simulink library "StateEstimation_lib"  (R2016b)
settings: Solver=VariableStepAuto  StartTime=0.0  StopTime=10.0  RelTol=1e-3
values from neighbouring files (symbols this model uses):
  accel_bias_init = zeros(3,1)    [Copy_of_StateEstimator_RIEKF.m]    (also in Quaternion_EKF.m; RightInvariant_EKF.m; StateEstimator_EKF.m; StateEstimator_RIEKF.m)
  accel_bias_noise_std = 0.1*ones(3,1)    [Copy_of_StateEstimator_RIEKF.m]    (also in Quaternion_EKF.m; RightInvariant_EKF.m; StateEstimator_EKF.m; StateEstimator_RIEKF.m)
  accel_noise_std = 0.1*ones(3,1)    [Copy_of_StateEstimator_RIEKF.m]    (also in Quaternion_EKF.m; RightInvariant_EKF.m; StateEstimator_EKF.m; StateEstimator_RIEKF.m)
  gyro_bias_init = zeros(3,1)    [Copy_of_StateEstimator_RIEKF.m]    (also in Quaternion_EKF.m; RightInvariant_EKF.m; StateEstimator_EKF.m; StateEstimator_RIEKF.m)
  gyro_bias_noise_std = 0.1*ones(3,1)    [Copy_of_StateEstimator_RIEKF.m]    (also in Quaternion_EKF.m; RightInvariant_EKF.m; StateEstimator_EKF.m; StateEstimator_RIEKF.m)
  gyro_noise_std = 0.1*ones(3,1)    [Copy_of_StateEstimator_RIEKF.m]    (also in Quaternion_EKF.m; RightInvariant_EKF.m; StateEstimator_EKF.m; StateEstimator_RIEKF.m)
undefined symbols (not defined in the file or in its folder): cassieParameters, CassieParameters, EKF_SampleTime, q_init, v_init
libraries: xpcutilitieslib x41, xpcrtudplib x41, dspfdesign x10, simulink x6, slrtlib x5
(part 2 of 4)

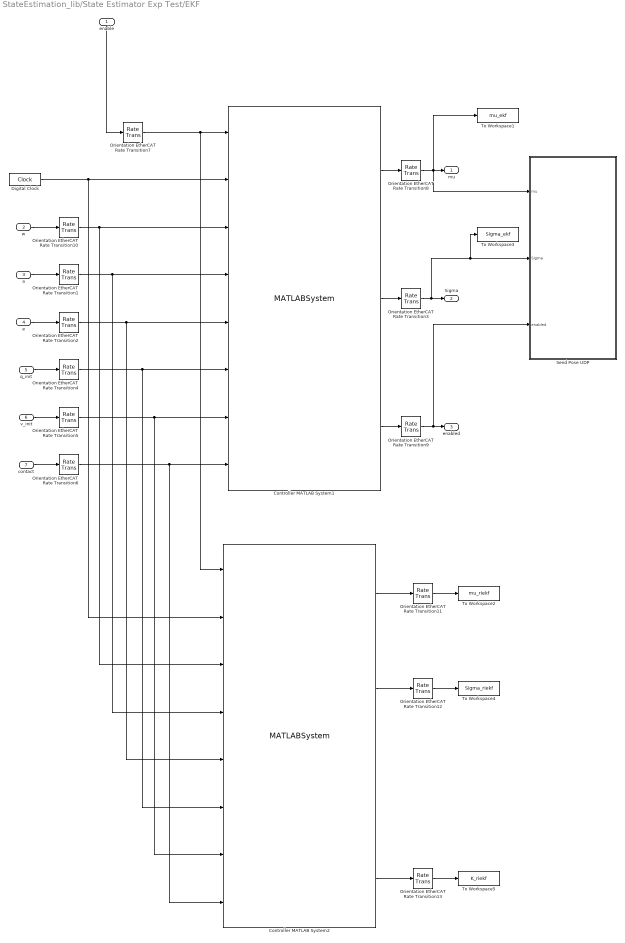
== system StateEstimation_lib/State Estimator Exp Test/EKF ==
  enable : Inport
  w : Inport  Port=2
  a : Inport  Port=3
  e : Inport  Port=4
  q_init : Inport  Port=5
  v_init : Inport  Port=6
  contact : Inport  Port=7
  Controller MATLAB System1 : MATLABSystem  System=StateEstimator_EKF  static_bias_initialization=static_bias_initialization  ekf_update_enabled=true  dt=EKF_SampleTime  enable_bias_estimation=enable_bias_estimation  gyro_noise_std=gyro_noise_std  gyro_bias_noise_std=gyro_bias_noise_std  accel_noise_std=accel_noise_std  accel_bias_noise_std=accel_bias_noise_std  contact_noise_std=contact_noise_std  encoder_noise_std=encoder_noise_std  gyro_bias_init=gyro_bias_init  accel_bias_init=accel_bias_init  SimulateUsing=Code generation
      mask Type: StateEstimator_EKF
      mask Display:
      | disp('StateEstimator_EKF');
      | port_label('input',1,'EnableFilter');
      | port_label('input',2,'t');
      | port_label('input',3,'w');
      | port_label('input',4,'a');
      | port_label('input',5,'e');
      | port_label('input',6,'q_init');
      | port_label('input',7,'v_init');
      | port_label('input',8,'contact');
      | port_label('output',1,'mu');
      | port_label('output',2,'Sigma');
      | port_label('output',3,'enabled');
  Controller MATLAB System2 : MATLABSystem  System=StateEstimator_RIEKF  static_bias_initialization=static_bias_initialization  ekf_update_enabled=true  dt=EKF_SampleTime  enable_bias_estimation=enable_bias_estimation  gyro_noise_std=gyro_noise_std  gyro_bias_noise_std=gyro_bias_noise_std  accel_noise_std=accel_noise_std  accel_bias_noise_std=accel_bias_noise_std  contact_noise_std=contact_noise_std  encoder_noise_std=encoder_noise_std  gyro_bias_init=gyro_bias_init  accel_bias_init=accel_bias_init  SimulateUsing=Code generation
      mask Type: StateEstimator_RIEKF
      mask Display:
      | disp('StateEstimator_RIEKF');
      | port_label('input',1,'EnableFilter');
      | port_label('input',2,'t');
      | port_label('input',3,'w');
      | port_label('input',4,'a');
      | port_label('input',5,'e');
      | port_label('input',6,'q_init');
      | port_label('input',7,'v_init');
      | port_label('input',8,'contact');
      | port_label('output',1,'mu');
      | port_label('output',2,'Sigma');
      | port_label('output',3,'enabled');
      | port_label('output',4,'K');
  Digital Clock : DigitalClock  SampleTime=EKF_SampleTime
  Orientation EtherCAT Rate Transition{1..2,4..7,10} (7 alike) : RateTransition  Deterministic=off  OutPortSampleTime=EKF_SampleTime
  Orientation EtherCAT Rate Transition{3,8..9,11..13} (6 alike) : RateTransition  Deterministic=off  OutPortSampleTime=CassieParameters.etherCatSampleTime
  Send Pose UDP : Subsystem
  To Workspace1 : ToWorkspace  VariableName=mu_ekf  SaveFormat=Timeseries  SampleTime=-1
  To Workspace2 : ToWorkspace  VariableName=mu_riekf  SaveFormat=Timeseries  SampleTime=-1
  To Workspace3 : ToWorkspace  VariableName=Sigma_ekf  SaveFormat=Timeseries  SampleTime=-1
  To Workspace4 : ToWorkspace  VariableName=Sigma_riekf  SaveFormat=Timeseries  SampleTime=-1
  To Workspace5 : ToWorkspace  VariableName=K_riekf  SaveFormat=Timeseries  SampleTime=-1
  mu : Outport
  Sigma : Outport  Port=2
  enabled : Outport  Port=3
  wires:
  enable/1 -> Orientation EtherCAT Rate Transition7/1
  Orientation EtherCAT Rate Transition7/1 -> Controller MATLAB System2/1, Controller MATLAB System1/1
  Orientation EtherCAT Rate Transition8/1 -> To Workspace1/1, Send Pose UDP/1(mu), mu/1
  Digital Clock/1 -> Controller MATLAB System2/2, Controller MATLAB System1/2
  Orientation EtherCAT Rate Transition9/1 -> Send Pose UDP/3(enabled), enabled/1
  Controller MATLAB System1/1 -> Orientation EtherCAT Rate Transition8/1
  Controller MATLAB System1/3 -> Orientation EtherCAT Rate Transition9/1
  Orientation EtherCAT Rate Transition6/1 -> Controller MATLAB System2/8, Controller MATLAB System1/8
  Orientation EtherCAT Rate Transition5/1 -> Controller MATLAB System2/7, Controller MATLAB System1/7
  q_init/1 -> Orientation EtherCAT Rate Transition4/1
  v_init/1 -> Orientation EtherCAT Rate Transition5/1
  contact/1 -> Orientation EtherCAT Rate Transition6/1
  w/1 -> Orientation EtherCAT Rate Transition10/1
  Orientation EtherCAT Rate Transition10/1 -> Controller MATLAB System2/3, Controller MATLAB System1/3
  a/1 -> Orientation EtherCAT Rate Transition1/1
  e/1 -> Orientation EtherCAT Rate Transition2/1
  Controller MATLAB System1/2 -> Orientation EtherCAT Rate Transition3/1
  Orientation EtherCAT Rate Transition3/1 -> To Workspace3/1, Send Pose UDP/2(Sigma), Sigma/1
  Orientation EtherCAT Rate Transition1/1 -> Controller MATLAB System2/4, Controller MATLAB System1/4
  Orientation EtherCAT Rate Transition2/1 -> Controller MATLAB System2/5, Controller MATLAB System1/5
  Orientation EtherCAT Rate Transition4/1 -> Controller MATLAB System2/6, Controller MATLAB System1/6
  Controller MATLAB System2/1 -> Orientation EtherCAT Rate Transition11/1
  Orientation EtherCAT Rate Transition11/1 -> To Workspace2/1
  Controller MATLAB System2/2 -> Orientation EtherCAT Rate Transition12/1
  Orientation EtherCAT Rate Transition12/1 -> To Workspace4/1
  Controller MATLAB System2/4 -> Orientation EtherCAT Rate Transition13/1
  Orientation EtherCAT Rate Transition13/1 -> To Workspace5/1

== system StateEstimation_lib/State Estimator Exp Test/Kinematic Velocity Estimator ==
  w : Inport
  q : Inport  Port=2
  dq : Inport  Port=3
  contact : Inport  Port=4
  Kinematic_Velocity : MATLAB Function  TreatAsAtomicUnit=on
  Selector2 : Selector  InputPortWidth=20  IndexOptions=Index vector (dialog)  Indices=[7:20]  OutputSizes=1
  Selector3 : Selector  InputPortWidth=20  IndexOptions=Index vector (dialog)  Indices=[7:20]  OutputSizes=1
  velocity_kinematic : Outport
  wires:
  w/1 -> Kinematic_Velocity/1(w)
  contact/1 -> Kinematic_Velocity/4(contact)
  dq/1 -> Selector3/1
  Kinematic_Velocity/1(velocity) -> velocity_kinematic/1
  q/1 -> Selector2/1
  Selector3/1 -> Kinematic_Velocity/3(e_dot)
  Selector2/1 -> Kinematic_Velocity/2(e)

== system StateEstimation_lib/State Estimator Exp Test/Local Map UDP ==
  note: Local Map UDP Data Structure
      |
      | Map Information
      | double time
      | double resolution
      | double length_x
      | double length_y
      |
      | Map Center Pose
      | double position_x
      | double position_y
      | double position_z
      | double orientation_x
      | double orientation_y
      | double orientation_z
      | double orientation_w
      |
      | Update Block Data
      | double row_start_index
      | double column_start_index
      | double[100] elevation_data
  "Byte Unpacking " : xpcutilitieslib/Byte Unpacking   MaskUnpackedDataTypes={'double'}  MaskUnpackedDataSizes={[45]}  MaskAlignment=1
  Data Store Memory : DataStoreMemory  DataStoreName=local_map  ReadBeforeWriteMsg=warning  WriteAfterWriteMsg=warning  WriteAfterReadMsg=warning  ShowAdditionalParam=off
  Data Store Write : DataStoreWrite  DataStoreName=local_map
  Receive : xpcrtudplib/UDP Receive  ipAddressVal=Use host-target connection  localPort=25000  rcvWidth=45*8  rcvFmAny=off  fmAddress=10.10.10.5  sampleTime=-1
  Terminator : Terminator
  wires:
  Receive/2 -> Terminator/1
  Receive/1 -> "Byte Unpacking "/1
  "Byte Unpacking "/1 -> Data Store Write/1

== system StateEstimation_lib/State Estimator Exp Test/Parse Outputs ==
  outputs : Inport
  Bus Selector : BusSelector  OutputSignals=radio
  Parse_Outputs : MATLAB Function  TreatAsAtomicUnit=on
  Send IMU UDP : Subsystem
  Send JointState UDP : Subsystem
  Send Radio : Subsystem
  Send Time : Subsystem
  qwi : Outport
  wi : Outport  Port=2
  ai : Outport  Port=3
  q : Outport  Port=4
  dq : Outport  Port=5
  wires:
  Bus Selector/1 -> Send Radio/1(radio)  "<radio>"
  Parse_Outputs/5(dq) -> dq/1, Send JointState UDP/2(dq)
  outputs/1 -> Bus Selector/1, Parse_Outputs/1(outputs)
  Parse_Outputs/2(wi) -> Send IMU UDP/2(w), wi/1
  Parse_Outputs/4(q) -> q/1, Send JointState UDP/1(q)
  Parse_Outputs/1(qwi) -> qwi/1, Send IMU UDP/1(q)
  Parse_Outputs/3(ai) -> Send IMU UDP/3(a), ai/1

== system StateEstimation_lib/State Estimator Exp Test/Reconstruct State ==
  q_in : Inport
  dq_in : Inport  Port=2
  w : Inport  Port=3
  contact : Inport  Port=4
  mu_in : Inport  Port=5
  ekf_enabled : Inport  Port=6
  Construct_State : MATLAB Function  TreatAsAtomicUnit=on
  Low Pass Filter : Subsystem  TreatAsAtomicUnit=on
  Mux : Mux
  Scope 6 : slrtlib/Displays and Logging/Scope   scopeno=2  scopetype=File  autostart=on  viewmode=Numerical  formatstr='%15.6f'  grid=on  ylimits=[0,0]  nosamples=250  noprepostsamples=0  interleave=1  triggermode=FreeRun  triggersignal=1  trigsignalfromport=on  triggerlevel=0.5  triggerslope=Rising  triggerscope=1  triggersample=0  filename=ekf1.dat  mode=Commit  writesize=512  autorestart=on  dynamicfilemode=off  maxwritefilesize=4000*1024^2
  q : Outport
  dq : Outport  Port=2
  velocity : Outport  Port=3
  wires:
  Low Pass Filter/1(filtered_signal) -> velocity/1
  mu_in/1 -> Construct_State/5(mu), Mux/3
  dq_in/1 -> Construct_State/2("dq ")
  Construct_State/1(q) -> q/1
  Construct_State/3(velocity) -> Mux/1, Low Pass Filter/1(signal)
  Construct_State/5(filter_selector) -> Low Pass Filter/2(selector)
  Mux/1 -> Scope 6/1
  q_in/1 -> Construct_State/1("q ")
  ekf_enabled/1 -> Construct_State/6(ekf_enabled), Mux/4
  Construct_State/2(dq) -> dq/1
  w/1 -> Construct_State/3(w)
  contact/1 -> Construct_State/4(contact)
  Construct_State/4(velocity_kinematic) -> Mux/2

== system StateEstimation_lib/State Estimator Sim Test/Contact Estimator ==
  q : Inport
  GRF_Estimator : MATLAB Function  TreatAsAtomicUnit=on
  Selector : Selector  InputPortWidth=4  IndexOptions=Index vector (dialog)  Indices=[2, 4]  OutputSizes=1
  Send Contact : Subsystem
  GRF : Outport
  contact : Outport  Port=2
  wires:
  GRF_Estimator/1(GRF) -> Selector/1, GRF/1
  GRF_Estimator/2(contact) -> contact/1
  q/1 -> GRF_Estimator/1(q)
  Selector/1 -> Send Contact/1(contact)

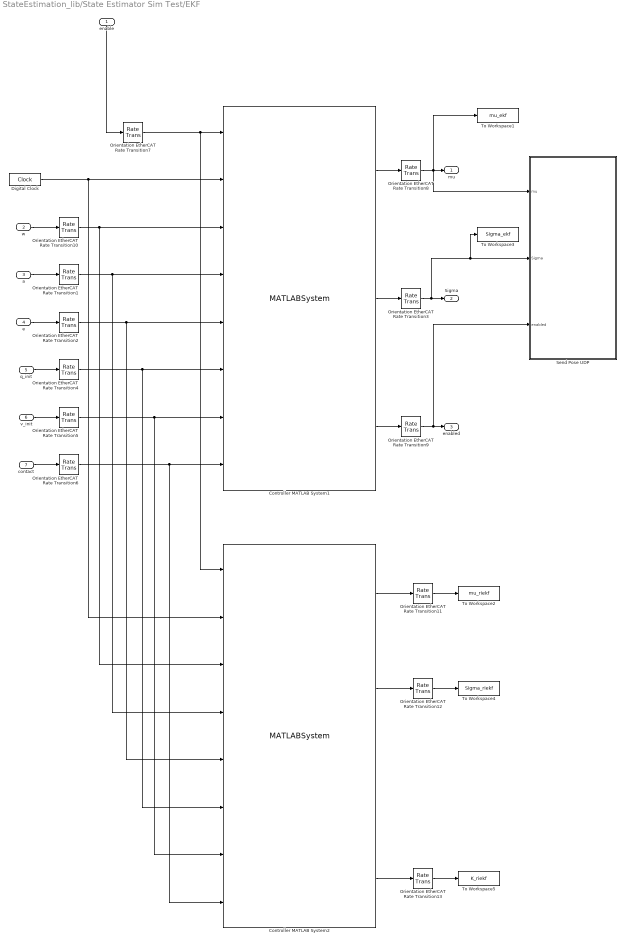
== system StateEstimation_lib/State Estimator Sim Test/EKF ==
  enable : Inport
  w : Inport  Port=2
  a : Inport  Port=3
  e : Inport  Port=4
  q_init : Inport  Port=5
  v_init : Inport  Port=6
  contact : Inport  Port=7
  Controller MATLAB System1 : MATLABSystem  System=StateEstimator_EKF  static_bias_initialization=true  ekf_update_enabled=true  dt=EKF_SampleTime  enable_bias_estimation=enable_bias_estimation  gyro_noise_std=gyro_noise_std  gyro_bias_noise_std=gyro_bias_noise_std  accel_noise_std=accel_noise_std  accel_bias_noise_std=accel_bias_noise_std  contact_noise_std=contact_noise_std  encoder_noise_std=encoder_noise_std  gyro_bias_init=[0;0;0]  accel_bias_init=[0;0;0]  SimulateUsing=Interpreted execution
      mask Type: StateEstimator_EKF
      mask Display:
      | disp('StateEstimator_EKF');
      | port_label('input',1,'EnableFilter');
      | port_label('input',2,'t');
      | port_label('input',3,'w');
      | port_label('input',4,'a');
      | port_label('input',5,'e');
      | port_label('input',6,'q_init');
      | port_label('input',7,'v_init');
      | port_label('input',8,'contact');
      | port_label('output',1,'mu');
      | port_label('output',2,'Sigma');
      | port_label('output',3,'enabled');
  Controller MATLAB System2 : MATLABSystem  System=StateEstimator_RIEKF  static_bias_initialization=true  ekf_update_enabled=true  dt=EKF_SampleTime  enable_bias_estimation=enable_bias_estimation  gyro_noise_std=gyro_noise_std  gyro_bias_noise_std=gyro_bias_noise_std  accel_noise_std=accel_noise_std  accel_bias_noise_std=accel_bias_noise_std  contact_noise_std=contact_noise_std  encoder_noise_std=encoder_noise_std  gyro_bias_init=[0;0;0]  accel_bias_init=[0;0;0]  SimulateUsing=Code generation
      mask Type: StateEstimator_RIEKF
      mask Display:
      | disp('StateEstimator_RIEKF');
      | port_label('input',1,'EnableFilter');
      | port_label('input',2,'t');
      | port_label('input',3,'w');
      | port_label('input',4,'a');
      | port_label('input',5,'e');
      | port_label('input',6,'q_init');
      | port_label('input',7,'v_init');
      | port_label('input',8,'contact');
      | port_label('output',1,'mu');
      | port_label('output',2,'Sigma');
      | port_label('output',3,'enabled');
      | port_label('output',4,'K');
  Digital Clock : DigitalClock  SampleTime=EKF_SampleTime
  Orientation EtherCAT Rate Transition{1..2,4..7,10} (7 alike) : RateTransition  Deterministic=off  OutPortSampleTime=EKF_SampleTime
  Orientation EtherCAT Rate Transition{3,8..9,11..13} (6 alike) : RateTransition  Deterministic=off  OutPortSampleTime=CassieParameters.etherCatSampleTime
  Send Pose UDP : Subsystem
  To Workspace1 : ToWorkspace  VariableName=mu_ekf  SaveFormat=Timeseries  SampleTime=-1
  To Workspace2 : ToWorkspace  VariableName=mu_riekf  SaveFormat=Timeseries  SampleTime=-1
  To Workspace3 : ToWorkspace  VariableName=Sigma_ekf  SaveFormat=Timeseries  SampleTime=-1
  To Workspace4 : ToWorkspace  VariableName=Sigma_riekf  SaveFormat=Timeseries  SampleTime=-1
  To Workspace5 : ToWorkspace  VariableName=K_riekf  SaveFormat=Timeseries  SampleTime=-1
  mu : Outport
  Sigma : Outport  Port=2
  enabled : Outport  Port=3
  wires:
  enable/1 -> Orientation EtherCAT Rate Transition7/1
  Orientation EtherCAT Rate Transition7/1 -> Controller MATLAB System2/1, Controller MATLAB System1/1
  Orientation EtherCAT Rate Transition8/1 -> To Workspace1/1, Send Pose UDP/1(mu), mu/1
  Digital Clock/1 -> Controller MATLAB System2/2, Controller MATLAB System1/2
  Orientation EtherCAT Rate Transition9/1 -> Send Pose UDP/3(enabled), enabled/1
  Controller MATLAB System1/1 -> Orientation EtherCAT Rate Transition8/1
  Controller MATLAB System1/3 -> Orientation EtherCAT Rate Transition9/1
  Orientation EtherCAT Rate Transition6/1 -> Controller MATLAB System2/8, Controller MATLAB System1/8
  Orientation EtherCAT Rate Transition5/1 -> Controller MATLAB System2/7, Controller MATLAB System1/7
  q_init/1 -> Orientation EtherCAT Rate Transition4/1
  v_init/1 -> Orientation EtherCAT Rate Transition5/1
  contact/1 -> Orientation EtherCAT Rate Transition6/1
  w/1 -> Orientation EtherCAT Rate Transition10/1
  Orientation EtherCAT Rate Transition10/1 -> Controller MATLAB System2/3, Controller MATLAB System1/3
  a/1 -> Orientation EtherCAT Rate Transition1/1
  e/1 -> Orientation EtherCAT Rate Transition2/1
  Controller MATLAB System1/2 -> Orientation EtherCAT Rate Transition3/1
  Orientation EtherCAT Rate Transition3/1 -> To Workspace3/1, Send Pose UDP/2(Sigma), Sigma/1
  Orientation EtherCAT Rate Transition1/1 -> Controller MATLAB System2/4, Controller MATLAB System1/4
  Orientation EtherCAT Rate Transition2/1 -> Controller MATLAB System2/5, Controller MATLAB System1/5
  Orientation EtherCAT Rate Transition4/1 -> Controller MATLAB System2/6, Controller MATLAB System1/6
  Controller MATLAB System2/1 -> Orientation EtherCAT Rate Transition11/1
  Orientation EtherCAT Rate Transition11/1 -> To Workspace2/1
  Controller MATLAB System2/2 -> Orientation EtherCAT Rate Transition12/1
  Orientation EtherCAT Rate Transition12/1 -> To Workspace4/1
  Controller MATLAB System2/4 -> Orientation EtherCAT Rate Transition13/1
  Orientation EtherCAT Rate Transition13/1 -> To Workspace5/1

== system StateEstimation_lib/State Estimator Sim Test/Kinematic Velocity Estimator ==
  w : Inport
  q : Inport  Port=2
  dq : Inport  Port=3
  contact : Inport  Port=4
  Kinematic_Velocity : MATLAB Function  TreatAsAtomicUnit=on
  Selector2 : Selector  InputPortWidth=20  IndexOptions=Index vector (dialog)  Indices=[7:20]  OutputSizes=1
  Selector3 : Selector  InputPortWidth=20  IndexOptions=Index vector (dialog)  Indices=[7:20]  OutputSizes=1
  velocity_kinematic : Outport
  wires:
  w/1 -> Kinematic_Velocity/1(w)
  contact/1 -> Kinematic_Velocity/4(contact)
  dq/1 -> Selector3/1
  Kinematic_Velocity/1(velocity) -> velocity_kinematic/1
  q/1 -> Selector2/1
  Selector3/1 -> Kinematic_Velocity/3(e_dot)
  Selector2/1 -> Kinematic_Velocity/2(e)

== system StateEstimation_lib/State Estimator Sim Test/Local Map UDP ==
  note: Local Map UDP Data Structure
      |
      | Map Information
      | double time
      | double resolution
      | double length_x
      | double length_y
      |
      | Map Center Pose
      | double position_x
      | double position_y
      | double position_z
      | double orientation_x
      | double orientation_y
      | double orientation_z
      | double orientation_w
      |
      | Update Block Data
      | double row_start_index
      | double column_start_index
      | double[100] elevation_data
  "Byte Unpacking " : xpcutilitieslib/Byte Unpacking   MaskUnpackedDataTypes={'double'}  MaskUnpackedDataSizes={[45]}  MaskAlignment=1
  Data Store Memory : DataStoreMemory  DataStoreName=local_map  ReadBeforeWriteMsg=warning  WriteAfterWriteMsg=warning  WriteAfterReadMsg=warning  ShowAdditionalParam=off
  Data Store Write : DataStoreWrite  DataStoreName=local_map
  Receive : xpcrtudplib/UDP Receive  ipAddressVal=Use host-target connection  localPort=25000  rcvWidth=45*8  rcvFmAny=off  fmAddress=10.10.10.5  sampleTime=-1
  Terminator : Terminator
  wires:
  Receive/2 -> Terminator/1
  Receive/1 -> "Byte Unpacking "/1
  "Byte Unpacking "/1 -> Data Store Write/1

== system StateEstimation_lib/State Estimator Sim Test/Parse Outputs ==
  outputs : Inport
  Bus Selector : BusSelector  OutputSignals=radio
  Parse_Outputs : MATLAB Function  TreatAsAtomicUnit=on
  Send IMU UDP : Subsystem
  Send JointState UDP : Subsystem
  Send Radio : Subsystem
  Send Time : Subsystem
  qwi : Outport
  wi : Outport  Port=2
  ai : Outport  Port=3
  q : Outport  Port=4
  dq : Outport  Port=5
  wires:
  Bus Selector/1 -> Send Radio/1(radio)  "<radio>"
  Parse_Outputs/5(dq) -> dq/1, Send JointState UDP/2(dq)
  outputs/1 -> Bus Selector/1, Parse_Outputs/1(outputs)
  Parse_Outputs/2(wi) -> Send IMU UDP/2(w), wi/1
  Parse_Outputs/4(q) -> q/1, Send JointState UDP/1(q)
  Parse_Outputs/1(qwi) -> qwi/1, Send IMU UDP/1(q)
  Parse_Outputs/3(ai) -> Send IMU UDP/3(a), ai/1

== system StateEstimation_lib/State Estimator Sim Test/Reconstruct State ==
  q_in : Inport
  dq_in : Inport  Port=2
  w : Inport  Port=3
  contact : Inport  Port=4
  mu_in : Inport  Port=5
  ekf_enabled : Inport  Port=6
  Construct_State : MATLAB Function  TreatAsAtomicUnit=on
  Low Pass Filter : Subsystem  TreatAsAtomicUnit=on
  Mux : Mux
  Scope 6 : slrtlib/Displays and Logging/Scope   scopeno=1  scopetype=File  autostart=on  viewmode=Numerical  formatstr='%15.6f'  grid=on  ylimits=[0,0]  nosamples=250  noprepostsamples=0  interleave=1  triggermode=FreeRun  triggersignal=1  trigsignalfromport=on  triggerlevel=0.5  triggerslope=Rising  triggerscope=1  triggersample=0  filename=ekf.dat  mode=Commit  writesize=512  autorestart=on  dynamicfilemode=off  maxwritefilesize=4000*1024^2
  q : Outport
  dq : Outport  Port=2
  velocity : Outport  Port=3
  wires:
  Low Pass Filter/1(filtered_signal) -> velocity/1
  mu_in/1 -> Construct_State/5(mu), Mux/3
  dq_in/1 -> Construct_State/2("dq ")
  Construct_State/1(q) -> q/1
  Construct_State/3(velocity) -> Mux/1, Low Pass Filter/1(signal)
  Construct_State/5(filter_selector) -> Low Pass Filter/2(selector)
  Mux/1 -> Scope 6/1
  q_in/1 -> Construct_State/1("q ")
  ekf_enabled/1 -> Construct_State/6(ekf_enabled), Mux/4
  Construct_State/2(dq) -> dq/1
  w/1 -> Construct_State/3(w)
  contact/1 -> Construct_State/4(contact)
  Construct_State/4(velocity_kinematic) -> Mux/2

== system StateEstimation_lib/Quaternion-based EKF/Contact Estimator/Send Contact ==
  contact : Inport
  "Byte Packing " : xpcutilitieslib/Byte Packing   MaskPackedDataType=uint8  MaskUnpackedDataTypes={'double'}  MaskAlignment=1
  Digital Clock : DigitalClock  SampleTime=CassieParameters.etherCatSampleTime
  Mux1 : Mux  Inputs=2
  Orientation EtherCAT Rate Transition10 : RateTransition  Deterministic=off  OutPortSampleTime=Contact_UDP_SampleTime
  Send : xpcrtudplib/UDP Send  ipAddressVal=Use host-target connection  localPort=-1  toAddress=10.10.10.5  toPort=25004  sampleTime=Contact_UDP_SampleTime
  Width : Width
  wires:
  Mux1/1 -> Orientation EtherCAT Rate Transition10/1
  "Byte Packing "/1 -> Width/1, Send/1
  Width/1 -> Send/2
  Orientation EtherCAT Rate Transition10/1 -> "Byte Packing "/1
  Digital Clock/1 -> Mux1/1
  contact/1 -> Mux1/2

== system StateEstimation_lib/Quaternion-based EKF/EKF/Send Pose UDP ==
  mu : Inport
  Sigma : Inport  Port=2
  enabled : Inport  Port=3
  "Byte Packing " : xpcutilitieslib/Byte Packing   MaskPackedDataType=uint8  MaskUnpackedDataTypes={'double'}  MaskAlignment=1
  ConstructPoseData : MATLAB Function  TreatAsAtomicUnit=on
  Digital Clock : DigitalClock  SampleTime=CassieParameters.etherCatSampleTime
  Mux1 : Mux
  Orientation EtherCAT Rate Transition10 : RateTransition  Deterministic=off  OutPortSampleTime=Pose_UDP_SampleTime
  Send : xpcrtudplib/UDP Send  ipAddressVal=Use host-target connection  localPort=-1  toAddress=10.10.10.5  toPort=25000  sampleTime=Pose_UDP_SampleTime
  Width : Width
  wires:
  Mux1/1 -> Orientation EtherCAT Rate Transition10/1
  "Byte Packing "/1 -> Width/1, Send/1
  Width/1 -> Send/2
  Orientation EtherCAT Rate Transition10/1 -> "Byte Packing "/1
  mu/1 -> Mux1/4, ConstructPoseData/1(mu)
  Sigma/1 -> ConstructPoseData/2(Sigma)
  enabled/1 -> Mux1/2
  Digital Clock/1 -> Mux1/1
  ConstructPoseData/1(pose_data) -> Mux1/3

== system StateEstimation_lib/Quaternion-based EKF/Parse Outputs/Send IMU UDP ==
  q : Inport
  w : Inport  Port=2
  a : Inport  Port=3
  "Byte Packing " : xpcutilitieslib/Byte Packing   MaskPackedDataType=uint8  MaskUnpackedDataTypes={'double'}  MaskAlignment=1
  Digital Clock : DigitalClock  SampleTime=CassieParameters.etherCatSampleTime
  Invert Quaterion for ROS : MATLAB Function  TreatAsAtomicUnit=on
  Mux1 : Mux
  Orientation EtherCAT Rate Transition10 : RateTransition  Deterministic=off  OutPortSampleTime=IMU_UDP_SampleTime
  Send : xpcrtudplib/UDP Send  ipAddressVal=Use host-target connection  localPort=-1  toAddress=10.10.10.5  toPort=25001  sampleTime=IMU_UDP_SampleTime
  Width : Width
  wires:
  Mux1/1 -> Orientation EtherCAT Rate Transition10/1
  "Byte Packing "/1 -> Width/1, Send/1
  Width/1 -> Send/2
  Orientation EtherCAT Rate Transition10/1 -> "Byte Packing "/1
  Digital Clock/1 -> Mux1/1
  a/1 -> Mux1/4
  q/1 -> Invert Quaterion for ROS/1(q)
  w/1 -> Mux1/3
  Invert Quaterion for ROS/1(q_inv) -> Mux1/2

== system StateEstimation_lib/Quaternion-based EKF/Parse Outputs/Send JointState UDP ==
  q : Inport
  dq : Inport  Port=2
  "Byte Packing " : xpcutilitieslib/Byte Packing   MaskPackedDataType=uint8  MaskUnpackedDataTypes={'double'}  MaskAlignment=1
  Digital Clock : DigitalClock  SampleTime=CassieParameters.etherCatSampleTime
  Mux1 : Mux  Inputs=3
  Orientation EtherCAT Rate Transition10 : RateTransition  Deterministic=off  OutPortSampleTime=JointState_UDP_SampleTime
  Parse_Outputs : MATLAB Function  TreatAsAtomicUnit=on
  Send : xpcrtudplib/UDP Send  ipAddressVal=Use host-target connection  localPort=-1  toAddress=10.10.10.5  toPort=25002  sampleTime=JointState_UDP_SampleTime
  Width : Width
  wires:
  Mux1/1 -> Orientation EtherCAT Rate Transition10/1
  "Byte Packing "/1 -> Width/1, Send/1
  Width/1 -> Send/2
  Orientation EtherCAT Rate Transition10/1 -> "Byte Packing "/1
  Digital Clock/1 -> Mux1/1
  Parse_Outputs/1(q_reduced) -> Mux1/2
  Parse_Outputs/2(dq_reduced) -> Mux1/3
  dq/1 -> Parse_Outputs/2(dq)
  q/1 -> Parse_Outputs/1(q)

== system StateEstimation_lib/Quaternion-based EKF/Parse Outputs/Send Radio ==
  radio : Inport
  "Byte Packing " : xpcutilitieslib/Byte Packing   MaskPackedDataType=uint8  MaskUnpackedDataTypes={'double'}  MaskAlignment=1
  Digital Clock : DigitalClock  SampleTime=CassieParameters.etherCatSampleTime
  Mux1 : Mux  Inputs=2
  Orientation EtherCAT Rate Transition10 : RateTransition  Deterministic=off  OutPortSampleTime=Radio_UDP_SampleTime
  Send : xpcrtudplib/UDP Send  ipAddressVal=Use host-target connection  localPort=-1  toAddress=10.10.10.5  toPort=25003  sampleTime=Radio_UDP_SampleTime
  Width : Width
  wires:
  Mux1/1 -> Orientation EtherCAT Rate Transition10/1
  "Byte Packing "/1 -> Width/1, Send/1
  Width/1 -> Send/2
  Orientation EtherCAT Rate Transition10/1 -> "Byte Packing "/1
  Digital Clock/1 -> Mux1/1
  radio/1 -> Mux1/2

== system StateEstimation_lib/Quaternion-based EKF/Parse Outputs/Send Time ==
  "Byte Packing " : xpcutilitieslib/Byte Packing   MaskPackedDataType=uint8  MaskUnpackedDataTypes={'double'}  MaskAlignment=1
  Digital Clock : DigitalClock  SampleTime=CassieParameters.etherCatSampleTime
  Orientation EtherCAT Rate Transition10 : RateTransition  Deterministic=off  OutPortSampleTime=Time_UDP_SampleTime
  Send : xpcrtudplib/UDP Send  ipAddressVal=Use host-target connection  localPort=-1  toAddress=10.10.10.105  toPort=25005  sampleTime=Time_UDP_SampleTime
  Width : Width
  wires:
  Digital Clock/1 -> Orientation EtherCAT Rate Transition10/1
  "Byte Packing "/1 -> Width/1, Send/1
  Width/1 -> Send/2
  Orientation EtherCAT Rate Transition10/1 -> "Byte Packing "/1

== system StateEstimation_lib/Quaternion-based EKF/Reconstruct State/Low Pass Filter ==
  signal : Inport  Partition=on  PartitionDimension=1  PartitionWidth=1
  selector : Inport  Port=2
  For Each : ForEach  DisableCoverage=on  IndexMode=One-based
  Lowpass Filter : dspfdesign/Lowpass Filter  FilterType=FIR  DesignForMinimumOrder=on  FilterOrder=50  PassbandFrequency=1  StopbandFrequency=10  PassbandRipple=1  StopbandAttenuation=20  InheritSampleRate=off  SampleRate=2000  SimulateUsing=Code generation  roundingMode=Floor  coeffsDataTypeStr=fixdt(1,16)
  Lowpass Filter1 : dspfdesign/Lowpass Filter  FilterType=FIR  DesignForMinimumOrder=on  FilterOrder=50  PassbandFrequency=1  StopbandFrequency=5  PassbandRipple=1  StopbandAttenuation=30  InheritSampleRate=off  SampleRate=2000  SimulateUsing=Code generation  roundingMode=Floor  coeffsDataTypeStr=fixdt(1,16)
  Switch : Switch  Criteria=u2 > Threshold
  filtered_signal : Outport  ConcatenationDimension=1
  wires:
  signal/1 -> Lowpass Filter1/1, Lowpass Filter/1
  selector/1 -> Switch/2
  Switch/1 -> filtered_signal/1
  Lowpass Filter/1 -> Switch/1
  Lowpass Filter1/1 -> Switch/3

== system StateEstimation_lib/Right-Invariant EKF/Contact Estimator/Send Contact ==
  contact : Inport
  "Byte Packing " : xpcutilitieslib/Byte Packing   MaskPackedDataType=uint8  MaskUnpackedDataTypes={'double'}  MaskAlignment=1
  Digital Clock : DigitalClock  SampleTime=CassieParameters.etherCatSampleTime
  Mux1 : Mux  Inputs=2
  Orientation EtherCAT Rate Transition10 : RateTransition  Deterministic=off  OutPortSampleTime=Contact_UDP_SampleTime
  Send : xpcrtudplib/UDP Send  ipAddressVal=Use host-target connection  localPort=-1  toAddress=10.10.10.5  toPort=25004  sampleTime=Contact_UDP_SampleTime
  Width : Width
  wires:
  Mux1/1 -> Orientation EtherCAT Rate Transition10/1
  "Byte Packing "/1 -> Width/1, Send/1
  Width/1 -> Send/2
  Orientation EtherCAT Rate Transition10/1 -> "Byte Packing "/1
  Digital Clock/1 -> Mux1/1
  contact/1 -> Mux1/2

== system StateEstimation_lib/Right-Invariant EKF/EKF/Send Pose UDP ==
  mu : Inport
  Sigma : Inport  Port=2
  enabled : Inport  Port=3
  "Byte Packing " : xpcutilitieslib/Byte Packing   MaskPackedDataType=uint8  MaskUnpackedDataTypes={'double'}  MaskAlignment=1
  ConstructPoseData : MATLAB Function  TreatAsAtomicUnit=on
  Digital Clock : DigitalClock  SampleTime=CassieParameters.etherCatSampleTime
  Mux1 : Mux
  Orientation EtherCAT Rate Transition10 : RateTransition  Deterministic=off  OutPortSampleTime=Pose_UDP_SampleTime
  Send : xpcrtudplib/UDP Send  ipAddressVal=Use host-target connection  localPort=-1  toAddress=10.10.10.5  toPort=25000  sampleTime=Pose_UDP_SampleTime
  Width : Width
  wires:
  Mux1/1 -> Orientation EtherCAT Rate Transition10/1
  "Byte Packing "/1 -> Width/1, Send/1
  Width/1 -> Send/2
  Orientation EtherCAT Rate Transition10/1 -> "Byte Packing "/1
  mu/1 -> Mux1/4, ConstructPoseData/1(mu)
  Sigma/1 -> ConstructPoseData/2(Sigma)
  enabled/1 -> Mux1/2
  Digital Clock/1 -> Mux1/1
  ConstructPoseData/1(pose_data) -> Mux1/3

== system StateEstimation_lib/Right-Invariant EKF/Parse Outputs/Send IMU UDP ==
  q : Inport
  w : Inport  Port=2
  a : Inport  Port=3
  "Byte Packing " : xpcutilitieslib/Byte Packing   MaskPackedDataType=uint8  MaskUnpackedDataTypes={'double'}  MaskAlignment=1
  Digital Clock : DigitalClock  SampleTime=CassieParameters.etherCatSampleTime
  Invert Quaterion for ROS : MATLAB Function  TreatAsAtomicUnit=on
  Mux1 : Mux
  Orientation EtherCAT Rate Transition10 : RateTransition  Deterministic=off  OutPortSampleTime=IMU_UDP_SampleTime
  Send : xpcrtudplib/UDP Send  ipAddressVal=Use host-target connection  localPort=-1  toAddress=10.10.10.5  toPort=25001  sampleTime=IMU_UDP_SampleTime
  Width : Width
  wires:
  Mux1/1 -> Orientation EtherCAT Rate Transition10/1
  "Byte Packing "/1 -> Width/1, Send/1
  Width/1 -> Send/2
  Orientation EtherCAT Rate Transition10/1 -> "Byte Packing "/1
  Digital Clock/1 -> Mux1/1
  a/1 -> Mux1/4
  q/1 -> Invert Quaterion for ROS/1(q)
  w/1 -> Mux1/3
  Invert Quaterion for ROS/1(q_inv) -> Mux1/2

== system StateEstimation_lib/Right-Invariant EKF/Parse Outputs/Send JointState UDP ==
  q : Inport
  dq : Inport  Port=2
  "Byte Packing " : xpcutilitieslib/Byte Packing   MaskPackedDataType=uint8  MaskUnpackedDataTypes={'double'}  MaskAlignment=1
  Digital Clock : DigitalClock  SampleTime=CassieParameters.etherCatSampleTime
  Mux1 : Mux  Inputs=3
  Orientation EtherCAT Rate Transition10 : RateTransition  Deterministic=off  OutPortSampleTime=JointState_UDP_SampleTime
  Parse_Outputs : MATLAB Function  TreatAsAtomicUnit=on
  Send : xpcrtudplib/UDP Send  ipAddressVal=Use host-target connection  localPort=-1  toAddress=10.10.10.5  toPort=25002  sampleTime=JointState_UDP_SampleTime
  Width : Width
  wires:
  Mux1/1 -> Orientation EtherCAT Rate Transition10/1
  "Byte Packing "/1 -> Width/1, Send/1
  Width/1 -> Send/2
  Orientation EtherCAT Rate Transition10/1 -> "Byte Packing "/1
  Digital Clock/1 -> Mux1/1
  Parse_Outputs/1(q_reduced) -> Mux1/2
  Parse_Outputs/2(dq_reduced) -> Mux1/3
  dq/1 -> Parse_Outputs/2(dq)
  q/1 -> Parse_Outputs/1(q)

== system StateEstimation_lib/Right-Invariant EKF/Parse Outputs/Send Radio ==
  radio : Inport
  "Byte Packing " : xpcutilitieslib/Byte Packing   MaskPackedDataType=uint8  MaskUnpackedDataTypes={'double'}  MaskAlignment=1
  Digital Clock : DigitalClock  SampleTime=CassieParameters.etherCatSampleTime
  Mux1 : Mux  Inputs=2
  Orientation EtherCAT Rate Transition10 : RateTransition  Deterministic=off  OutPortSampleTime=Radio_UDP_SampleTime
  Send : xpcrtudplib/UDP Send  ipAddressVal=Use host-target connection  localPort=-1  toAddress=10.10.10.5  toPort=25003  sampleTime=Radio_UDP_SampleTime
  Width : Width
  wires:
  Mux1/1 -> Orientation EtherCAT Rate Transition10/1
  "Byte Packing "/1 -> Width/1, Send/1
  Width/1 -> Send/2
  Orientation EtherCAT Rate Transition10/1 -> "Byte Packing "/1
  Digital Clock/1 -> Mux1/1
  radio/1 -> Mux1/2

== system StateEstimation_lib/Right-Invariant EKF/Parse Outputs/Send Time ==
  "Byte Packing " : xpcutilitieslib/Byte Packing   MaskPackedDataType=uint8  MaskUnpackedDataTypes={'double'}  MaskAlignment=1
  Digital Clock : DigitalClock  SampleTime=CassieParameters.etherCatSampleTime
  Orientation EtherCAT Rate Transition10 : RateTransition  Deterministic=off  OutPortSampleTime=Time_UDP_SampleTime
  Send : xpcrtudplib/UDP Send  ipAddressVal=Use host-target connection  localPort=-1  toAddress=10.10.10.105  toPort=25005  sampleTime=Time_UDP_SampleTime
  Width : Width
  wires:
  Digital Clock/1 -> Orientation EtherCAT Rate Transition10/1
  "Byte Packing "/1 -> Width/1, Send/1
  Width/1 -> Send/2
  Orientation EtherCAT Rate Transition10/1 -> "Byte Packing "/1

== system StateEstimation_lib/Right-Invariant EKF/Reconstruct State/Low Pass Filter ==
  signal : Inport  Partition=on  PartitionDimension=1  PartitionWidth=1
  selector : Inport  Port=2
  For Each : ForEach  DisableCoverage=on  IndexMode=One-based
  Lowpass Filter : dspfdesign/Lowpass Filter  FilterType=FIR  DesignForMinimumOrder=on  FilterOrder=50  PassbandFrequency=1  StopbandFrequency=10  PassbandRipple=1  StopbandAttenuation=20  InheritSampleRate=off  SampleRate=2000  SimulateUsing=Code generation  roundingMode=Floor  coeffsDataTypeStr=fixdt(1,16)
  Lowpass Filter1 : dspfdesign/Lowpass Filter  FilterType=FIR  DesignForMinimumOrder=on  FilterOrder=50  PassbandFrequency=1  StopbandFrequency=5  PassbandRipple=1  StopbandAttenuation=30  InheritSampleRate=off  SampleRate=2000  SimulateUsing=Code generation  roundingMode=Floor  coeffsDataTypeStr=fixdt(1,16)
  Switch : Switch  Criteria=u2 > Threshold
  filtered_signal : Outport  ConcatenationDimension=1
  wires:
  signal/1 -> Lowpass Filter1/1, Lowpass Filter/1
  selector/1 -> Switch/2
  Switch/1 -> filtered_signal/1
  Lowpass Filter/1 -> Switch/1
  Lowpass Filter1/1 -> Switch/3

== system StateEstimation_lib/Send UDP Only/Contact Estimator/Send Contact ==
  contact : Inport
  "Byte Packing " : xpcutilitieslib/Byte Packing   MaskPackedDataType=uint8  MaskUnpackedDataTypes={'double'}  MaskAlignment=1
  Digital Clock : DigitalClock  SampleTime=CassieParameters.etherCatSampleTime
  Mux1 : Mux  Inputs=2
  Orientation EtherCAT Rate Transition10 : RateTransition  Deterministic=off  OutPortSampleTime=Contact_UDP_SampleTime
  Send : xpcrtudplib/UDP Send  ipAddressVal=Use host-target connection  localPort=-1  toAddress=10.10.10.5  toPort=25004  sampleTime=Contact_UDP_SampleTime
  Width : Width
  wires:
  Mux1/1 -> Orientation EtherCAT Rate Transition10/1
  "Byte Packing "/1 -> Width/1, Send/1
  Width/1 -> Send/2
  Orientation EtherCAT Rate Transition10/1 -> "Byte Packing "/1
  Digital Clock/1 -> Mux1/1
  contact/1 -> Mux1/2

== system StateEstimation_lib/Send UDP Only/Parse Outputs/Send IMU UDP ==
  q : Inport
  w : Inport  Port=2
  a : Inport  Port=3
  "Byte Packing " : xpcutilitieslib/Byte Packing   MaskPackedDataType=uint8  MaskUnpackedDataTypes={'double'}  MaskAlignment=1
  Digital Clock : DigitalClock  SampleTime=CassieParameters.etherCatSampleTime
  Invert Quaterion for ROS : MATLAB Function  TreatAsAtomicUnit=on
  Mux1 : Mux
  Orientation EtherCAT Rate Transition10 : RateTransition  Deterministic=off  OutPortSampleTime=IMU_UDP_SampleTime
  Send : xpcrtudplib/UDP Send  ipAddressVal=Use host-target connection  localPort=-1  toAddress=10.10.10.5  toPort=25001  sampleTime=IMU_UDP_SampleTime
  Width : Width
  wires:
  Mux1/1 -> Orientation EtherCAT Rate Transition10/1
  "Byte Packing "/1 -> Width/1, Send/1
  Width/1 -> Send/2
  Orientation EtherCAT Rate Transition10/1 -> "Byte Packing "/1
  Digital Clock/1 -> Mux1/1
  a/1 -> Mux1/4
  q/1 -> Invert Quaterion for ROS/1(q)
  w/1 -> Mux1/3
  Invert Quaterion for ROS/1(q_inv) -> Mux1/2

== system StateEstimation_lib/Send UDP Only/Parse Outputs/Send JointState UDP ==
  q : Inport
  dq : Inport  Port=2
  "Byte Packing " : xpcutilitieslib/Byte Packing   MaskPackedDataType=uint8  MaskUnpackedDataTypes={'double'}  MaskAlignment=1
  Digital Clock : DigitalClock  SampleTime=CassieParameters.etherCatSampleTime
  Mux1 : Mux  Inputs=3
  Orientation EtherCAT Rate Transition10 : RateTransition  Deterministic=off  OutPortSampleTime=JointState_UDP_SampleTime
  Parse_Outputs : MATLAB Function  TreatAsAtomicUnit=on
  Send : xpcrtudplib/UDP Send  ipAddressVal=Use host-target connection  localPort=-1  toAddress=10.10.10.5  toPort=25002  sampleTime=JointState_UDP_SampleTime
  Width : Width
  wires:
  Mux1/1 -> Orientation EtherCAT Rate Transition10/1
  "Byte Packing "/1 -> Width/1, Send/1
  Width/1 -> Send/2
  Orientation EtherCAT Rate Transition10/1 -> "Byte Packing "/1
  Digital Clock/1 -> Mux1/1
  Parse_Outputs/1(q_reduced) -> Mux1/2
  Parse_Outputs/2(dq_reduced) -> Mux1/3
  dq/1 -> Parse_Outputs/2(dq)
  q/1 -> Parse_Outputs/1(q)

== system StateEstimation_lib/Send UDP Only/Parse Outputs/Send Radio ==
  radio : Inport
  "Byte Packing " : xpcutilitieslib/Byte Packing   MaskPackedDataType=uint8  MaskUnpackedDataTypes={'double'}  MaskAlignment=1
  Digital Clock : DigitalClock  SampleTime=CassieParameters.etherCatSampleTime
  Mux1 : Mux  Inputs=2
  Orientation EtherCAT Rate Transition10 : RateTransition  Deterministic=off  OutPortSampleTime=Radio_UDP_SampleTime
  Send : xpcrtudplib/UDP Send  ipAddressVal=Use host-target connection  localPort=-1  toAddress=10.10.10.5  toPort=25003  sampleTime=Radio_UDP_SampleTime
  Width : Width
  wires:
  Mux1/1 -> Orientation EtherCAT Rate Transition10/1
  "Byte Packing "/1 -> Width/1, Send/1
  Width/1 -> Send/2
  Orientation EtherCAT Rate Transition10/1 -> "Byte Packing "/1
  Digital Clock/1 -> Mux1/1
  radio/1 -> Mux1/2

== system StateEstimation_lib/Send UDP Only/Parse Outputs/Send Time ==
  "Byte Packing " : xpcutilitieslib/Byte Packing   MaskPackedDataType=uint8  MaskUnpackedDataTypes={'double'}  MaskAlignment=1
  Digital Clock : DigitalClock  SampleTime=CassieParameters.etherCatSampleTime
  Orientation EtherCAT Rate Transition10 : RateTransition  Deterministic=off  OutPortSampleTime=Time_UDP_SampleTime
  Send : xpcrtudplib/UDP Send  ipAddressVal=Use host-target connection  localPort=-1  toAddress=10.10.10.5  toPort=25005  sampleTime=Time_UDP_SampleTime
  Width : Width
  wires:
  Digital Clock/1 -> Orientation EtherCAT Rate Transition10/1
  "Byte Packing "/1 -> Width/1, Send/1
  Width/1 -> Send/2
  Orientation EtherCAT Rate Transition10/1 -> "Byte Packing "/1

== system StateEstimation_lib/State Estimator/Contact Estimator/Send Contact ==
  contact : Inport
  "Byte Packing " : xpcutilitieslib/Byte Packing   MaskPackedDataType=uint8  MaskUnpackedDataTypes={'double'}  MaskAlignment=1
  Digital Clock : DigitalClock  SampleTime=CassieParameters.etherCatSampleTime
  Mux1 : Mux  Inputs=2
  Orientation EtherCAT Rate Transition10 : RateTransition  Deterministic=off  OutPortSampleTime=Contact_UDP_SampleTime
  Send : xpcrtudplib/UDP Send  ipAddressVal=Use host-target connection  localPort=-1  toAddress=10.10.10.5  toPort=25004  sampleTime=Contact_UDP_SampleTime
  Width : Width
  wires:
  Mux1/1 -> Orientation EtherCAT Rate Transition10/1
  "Byte Packing "/1 -> Width/1, Send/1
  Width/1 -> Send/2
  Orientation EtherCAT Rate Transition10/1 -> "Byte Packing "/1
  Digital Clock/1 -> Mux1/1
  contact/1 -> Mux1/2

== system StateEstimation_lib/State Estimator/EKF/Send Pose UDP ==
  mu : Inport
  Sigma : Inport  Port=2
  enabled : Inport  Port=3
  "Byte Packing " : xpcutilitieslib/Byte Packing   MaskPackedDataType=uint8  MaskUnpackedDataTypes={'double'}  MaskAlignment=1
  ConstructPoseData : MATLAB Function  TreatAsAtomicUnit=on
  Digital Clock : DigitalClock  SampleTime=CassieParameters.etherCatSampleTime
  Mux1 : Mux
  Orientation EtherCAT Rate Transition10 : RateTransition  Deterministic=off  OutPortSampleTime=Pose_UDP_SampleTime
  Send : xpcrtudplib/UDP Send  ipAddressVal=Use host-target connection  localPort=-1  toAddress=10.10.10.5  toPort=25000  sampleTime=Pose_UDP_SampleTime
  Width : Width
  wires:
  Mux1/1 -> Orientation EtherCAT Rate Transition10/1
  "Byte Packing "/1 -> Width/1, Send/1
  Width/1 -> Send/2
  Orientation EtherCAT Rate Transition10/1 -> "Byte Packing "/1
  mu/1 -> Mux1/4, ConstructPoseData/1(mu)
  Sigma/1 -> ConstructPoseData/2(Sigma)
  enabled/1 -> Mux1/2
  Digital Clock/1 -> Mux1/1
  ConstructPoseData/1(pose_data) -> Mux1/3

== system StateEstimation_lib/State Estimator/Parse Outputs/Send IMU UDP ==
  q : Inport
  w : Inport  Port=2
  a : Inport  Port=3
  "Byte Packing " : xpcutilitieslib/Byte Packing   MaskPackedDataType=uint8  MaskUnpackedDataTypes={'double'}  MaskAlignment=1
  Digital Clock : DigitalClock  SampleTime=CassieParameters.etherCatSampleTime
  Invert Quaterion for ROS : MATLAB Function  TreatAsAtomicUnit=on
  Mux1 : Mux
  Orientation EtherCAT Rate Transition10 : RateTransition  Deterministic=off  OutPortSampleTime=IMU_UDP_SampleTime
  Send : xpcrtudplib/UDP Send  ipAddressVal=Use host-target connection  localPort=-1  toAddress=10.10.10.5  toPort=25001  sampleTime=IMU_UDP_SampleTime
  Width : Width
  wires:
  Mux1/1 -> Orientation EtherCAT Rate Transition10/1
  "Byte Packing "/1 -> Width/1, Send/1
  Width/1 -> Send/2
  Orientation EtherCAT Rate Transition10/1 -> "Byte Packing "/1
  Digital Clock/1 -> Mux1/1
  a/1 -> Mux1/4
  q/1 -> Invert Quaterion for ROS/1(q)
  w/1 -> Mux1/3
  Invert Quaterion for ROS/1(q_inv) -> Mux1/2

== system StateEstimation_lib/State Estimator/Parse Outputs/Send JointState UDP ==
  q : Inport
  dq : Inport  Port=2
  "Byte Packing " : xpcutilitieslib/Byte Packing   MaskPackedDataType=uint8  MaskUnpackedDataTypes={'double'}  MaskAlignment=1
  Digital Clock : DigitalClock  SampleTime=CassieParameters.etherCatSampleTime
  Mux1 : Mux  Inputs=3
  Orientation EtherCAT Rate Transition10 : RateTransition  Deterministic=off  OutPortSampleTime=JointState_UDP_SampleTime
  Parse_Outputs : MATLAB Function  TreatAsAtomicUnit=on
  Send : xpcrtudplib/UDP Send  ipAddressVal=Use host-target connection  localPort=-1  toAddress=10.10.10.5  toPort=25002  sampleTime=JointState_UDP_SampleTime
  Width : Width
  wires:
  Mux1/1 -> Orientation EtherCAT Rate Transition10/1
  "Byte Packing "/1 -> Width/1, Send/1
  Width/1 -> Send/2
  Orientation EtherCAT Rate Transition10/1 -> "Byte Packing "/1
  Digital Clock/1 -> Mux1/1
  Parse_Outputs/1(q_reduced) -> Mux1/2
  Parse_Outputs/2(dq_reduced) -> Mux1/3
  dq/1 -> Parse_Outputs/2(dq)
  q/1 -> Parse_Outputs/1(q)

== system StateEstimation_lib/State Estimator/Parse Outputs/Send Radio ==
  radio : Inport
  "Byte Packing " : xpcutilitieslib/Byte Packing   MaskPackedDataType=uint8  MaskUnpackedDataTypes={'double'}  MaskAlignment=1
  Digital Clock : DigitalClock  SampleTime=CassieParameters.etherCatSampleTime
  Mux1 : Mux  Inputs=2
  Orientation EtherCAT Rate Transition10 : RateTransition  Deterministic=off  OutPortSampleTime=Radio_UDP_SampleTime
  Send : xpcrtudplib/UDP Send  ipAddressVal=Use host-target connection  localPort=-1  toAddress=10.10.10.5  toPort=25003  sampleTime=Radio_UDP_SampleTime
  Width : Width
  wires:
  Mux1/1 -> Orientation EtherCAT Rate Transition10/1
  "Byte Packing "/1 -> Width/1, Send/1
  Width/1 -> Send/2
  Orientation EtherCAT Rate Transition10/1 -> "Byte Packing "/1
  Digital Clock/1 -> Mux1/1
  radio/1 -> Mux1/2

== system StateEstimation_lib/State Estimator/Parse Outputs/Send Time ==
  "Byte Packing " : xpcutilitieslib/Byte Packing   MaskPackedDataType=uint8  MaskUnpackedDataTypes={'double'}  MaskAlignment=1
  Digital Clock : DigitalClock  SampleTime=CassieParameters.etherCatSampleTime
  Orientation EtherCAT Rate Transition10 : RateTransition  Deterministic=off  OutPortSampleTime=Time_UDP_SampleTime
  Send : xpcrtudplib/UDP Send  ipAddressVal=Use host-target connection  localPort=-1  toAddress=10.10.10.105  toPort=25005  sampleTime=Time_UDP_SampleTime
  Width : Width
  wires:
  Digital Clock/1 -> Orientation EtherCAT Rate Transition10/1
  "Byte Packing "/1 -> Width/1, Send/1
  Width/1 -> Send/2
  Orientation EtherCAT Rate Transition10/1 -> "Byte Packing "/1

== system StateEstimation_lib/State Estimator/Reconstruct State/Low Pass Filter ==
  signal : Inport  Partition=on  PartitionDimension=1  PartitionWidth=1
  selector : Inport  Port=2
  For Each : ForEach  DisableCoverage=on  IndexMode=One-based
  Lowpass Filter : dspfdesign/Lowpass Filter  FilterType=FIR  DesignForMinimumOrder=on  FilterOrder=50  PassbandFrequency=1  StopbandFrequency=10  PassbandRipple=1  StopbandAttenuation=20  InheritSampleRate=off  SampleRate=2000  SimulateUsing=Code generation  roundingMode=Floor  coeffsDataTypeStr=fixdt(1,16)
  Lowpass Filter1 : dspfdesign/Lowpass Filter  FilterType=FIR  DesignForMinimumOrder=on  FilterOrder=50  PassbandFrequency=1  StopbandFrequency=5  PassbandRipple=1  StopbandAttenuation=30  InheritSampleRate=off  SampleRate=2000  SimulateUsing=Code generation  roundingMode=Floor  coeffsDataTypeStr=fixdt(1,16)
  Switch : Switch  Criteria=u2 > Threshold
  filtered_signal : Outport  ConcatenationDimension=1
  wires:
  signal/1 -> Lowpass Filter1/1, Lowpass Filter/1
  selector/1 -> Switch/2
  Switch/1 -> filtered_signal/1
  Lowpass Filter/1 -> Switch/1
  Lowpass Filter1/1 -> Switch/3

== system StateEstimation_lib/State Estimator Exp Test/Contact Estimator/Send Contact ==
  contact : Inport
  "Byte Packing " : xpcutilitieslib/Byte Packing   MaskPackedDataType=uint8  MaskUnpackedDataTypes={'double'}  MaskAlignment=1
  Digital Clock : DigitalClock  SampleTime=CassieParameters.etherCatSampleTime
  Mux1 : Mux  Inputs=2
  Orientation EtherCAT Rate Transition10 : RateTransition  Deterministic=off  OutPortSampleTime=Contact_UDP_SampleTime
  Send : xpcrtudplib/UDP Send  ipAddressVal=Use host-target connection  localPort=-1  toAddress=10.10.10.5  toPort=25004  sampleTime=Contact_UDP_SampleTime
  Width : Width
  wires:
  Mux1/1 -> Orientation EtherCAT Rate Transition10/1
  "Byte Packing "/1 -> Width/1, Send/1
  Width/1 -> Send/2
  Orientation EtherCAT Rate Transition10/1 -> "Byte Packing "/1
  Digital Clock/1 -> Mux1/1
  contact/1 -> Mux1/2

== system StateEstimation_lib/State Estimator Exp Test/EKF/Send Pose UDP ==
  mu : Inport
  Sigma : Inport  Port=2
  enabled : Inport  Port=3
  "Byte Packing " : xpcutilitieslib/Byte Packing   MaskPackedDataType=uint8  MaskUnpackedDataTypes={'double'}  MaskAlignment=1
  ConstructPoseData : MATLAB Function  TreatAsAtomicUnit=on
  Digital Clock : DigitalClock  SampleTime=CassieParameters.etherCatSampleTime
  Mux1 : Mux
  Orientation EtherCAT Rate Transition10 : RateTransition  Deterministic=off  OutPortSampleTime=Pose_UDP_SampleTime
  Send : xpcrtudplib/UDP Send  ipAddressVal=Use host-target connection  localPort=-1  toAddress=10.10.10.5  toPort=25000  sampleTime=Pose_UDP_SampleTime
  Width : Width
  wires:
  Mux1/1 -> Orientation EtherCAT Rate Transition10/1
  "Byte Packing "/1 -> Width/1, Send/1
  Width/1 -> Send/2
  Orientation EtherCAT Rate Transition10/1 -> "Byte Packing "/1
  mu/1 -> Mux1/4, ConstructPoseData/1(mu)
  Sigma/1 -> ConstructPoseData/2(Sigma)
  enabled/1 -> Mux1/2
  Digital Clock/1 -> Mux1/1
  ConstructPoseData/1(pose_data) -> Mux1/3

== system StateEstimation_lib/State Estimator Exp Test/Parse Outputs/Send IMU UDP ==
  q : Inport
  w : Inport  Port=2
  a : Inport  Port=3
  "Byte Packing " : xpcutilitieslib/Byte Packing   MaskPackedDataType=uint8  MaskUnpackedDataTypes={'double'}  MaskAlignment=1
  Digital Clock : DigitalClock  SampleTime=CassieParameters.etherCatSampleTime
  Invert Quaterion for ROS : MATLAB Function  TreatAsAtomicUnit=on
  Mux1 : Mux
  Orientation EtherCAT Rate Transition10 : RateTransition  Deterministic=off  OutPortSampleTime=IMU_UDP_SampleTime
  Send : xpcrtudplib/UDP Send  ipAddressVal=Use host-target connection  localPort=-1  toAddress=10.10.10.5  toPort=25001  sampleTime=IMU_UDP_SampleTime
  Width : Width
  wires:
  Mux1/1 -> Orientation EtherCAT Rate Transition10/1
  "Byte Packing "/1 -> Width/1, Send/1
  Width/1 -> Send/2
  Orientation EtherCAT Rate Transition10/1 -> "Byte Packing "/1
  Digital Clock/1 -> Mux1/1
  a/1 -> Mux1/4
  q/1 -> Invert Quaterion for ROS/1(q)
  w/1 -> Mux1/3
  Invert Quaterion for ROS/1(q_inv) -> Mux1/2

== system StateEstimation_lib/State Estimator Exp Test/Parse Outputs/Send JointState UDP ==
  q : Inport
  dq : Inport  Port=2
  "Byte Packing " : xpcutilitieslib/Byte Packing   MaskPackedDataType=uint8  MaskUnpackedDataTypes={'double'}  MaskAlignment=1
  Digital Clock : DigitalClock  SampleTime=CassieParameters.etherCatSampleTime
  Mux1 : Mux  Inputs=3
  Orientation EtherCAT Rate Transition10 : RateTransition  Deterministic=off  OutPortSampleTime=JointState_UDP_SampleTime
  Parse_Outputs : MATLAB Function  TreatAsAtomicUnit=on
  Send : xpcrtudplib/UDP Send  ipAddressVal=Use host-target connection  localPort=-1  toAddress=10.10.10.5  toPort=25002  sampleTime=JointState_UDP_SampleTime
  Width : Width
  wires:
  Mux1/1 -> Orientation EtherCAT Rate Transition10/1
  "Byte Packing "/1 -> Width/1, Send/1
  Width/1 -> Send/2
  Orientation EtherCAT Rate Transition10/1 -> "Byte Packing "/1
  Digital Clock/1 -> Mux1/1
  Parse_Outputs/1(q_reduced) -> Mux1/2
  Parse_Outputs/2(dq_reduced) -> Mux1/3
  dq/1 -> Parse_Outputs/2(dq)
  q/1 -> Parse_Outputs/1(q)

== system StateEstimation_lib/State Estimator Exp Test/Parse Outputs/Send Radio ==
  radio : Inport
  "Byte Packing " : xpcutilitieslib/Byte Packing   MaskPackedDataType=uint8  MaskUnpackedDataTypes={'double'}  MaskAlignment=1
  Digital Clock : DigitalClock  SampleTime=CassieParameters.etherCatSampleTime
  Mux1 : Mux  Inputs=2
  Orientation EtherCAT Rate Transition10 : RateTransition  Deterministic=off  OutPortSampleTime=Radio_UDP_SampleTime
  Send : xpcrtudplib/UDP Send  ipAddressVal=Use host-target connection  localPort=-1  toAddress=10.10.10.5  toPort=25003  sampleTime=Radio_UDP_SampleTime
  Width : Width
  wires:
  Mux1/1 -> Orientation EtherCAT Rate Transition10/1
  "Byte Packing "/1 -> Width/1, Send/1
  Width/1 -> Send/2
  Orientation EtherCAT Rate Transition10/1 -> "Byte Packing "/1
  Digital Clock/1 -> Mux1/1
  radio/1 -> Mux1/2

== system StateEstimation_lib/State Estimator Exp Test/Parse Outputs/Send Time ==
  "Byte Packing " : xpcutilitieslib/Byte Packing   MaskPackedDataType=uint8  MaskUnpackedDataTypes={'double'}  MaskAlignment=1
  Digital Clock : DigitalClock  SampleTime=CassieParameters.etherCatSampleTime
  Orientation EtherCAT Rate Transition10 : RateTransition  Deterministic=off  OutPortSampleTime=Time_UDP_SampleTime
  Send : xpcrtudplib/UDP Send  ipAddressVal=Use host-target connection  localPort=-1  toAddress=10.10.10.105  toPort=25005  sampleTime=Time_UDP_SampleTime
  Width : Width
  wires:
  Digital Clock/1 -> Orientation EtherCAT Rate Transition10/1
  "Byte Packing "/1 -> Width/1, Send/1
  Width/1 -> Send/2
  Orientation EtherCAT Rate Transition10/1 -> "Byte Packing "/1

== system StateEstimation_lib/State Estimator Exp Test/Reconstruct State/Low Pass Filter ==
  signal : Inport  Partition=on  PartitionDimension=1  PartitionWidth=1
  selector : Inport  Port=2
  For Each : ForEach  DisableCoverage=on  IndexMode=One-based
  Lowpass Filter : dspfdesign/Lowpass Filter  FilterType=FIR  DesignForMinimumOrder=on  FilterOrder=50  PassbandFrequency=1  StopbandFrequency=10  PassbandRipple=1  StopbandAttenuation=20  InheritSampleRate=off  SampleRate=2000  SimulateUsing=Code generation  roundingMode=Floor  coeffsDataTypeStr=fixdt(1,16)
  Lowpass Filter1 : dspfdesign/Lowpass Filter  FilterType=FIR  DesignForMinimumOrder=on  FilterOrder=50  PassbandFrequency=1  StopbandFrequency=5  PassbandRipple=1  StopbandAttenuation=30  InheritSampleRate=off  SampleRate=2000  SimulateUsing=Code generation  roundingMode=Floor  coeffsDataTypeStr=fixdt(1,16)
  Switch : Switch  Criteria=u2 > Threshold
  filtered_signal : Outport  ConcatenationDimension=1
  wires:
  signal/1 -> Lowpass Filter1/1, Lowpass Filter/1
  selector/1 -> Switch/2
  Switch/1 -> filtered_signal/1
  Lowpass Filter/1 -> Switch/1
  Lowpass Filter1/1 -> Switch/3
